simulink model "lab08_3d"  (R2024b)
settings: Solver=ode45  StartTime=0.0  StopTime=15  MaxStep=0.02  MinStep=0.01  RelTol=1e-3
settings Model: Creator=kg53848  LastModifiedBy=kg53848
settings SolverCC: InitialStep=0.01

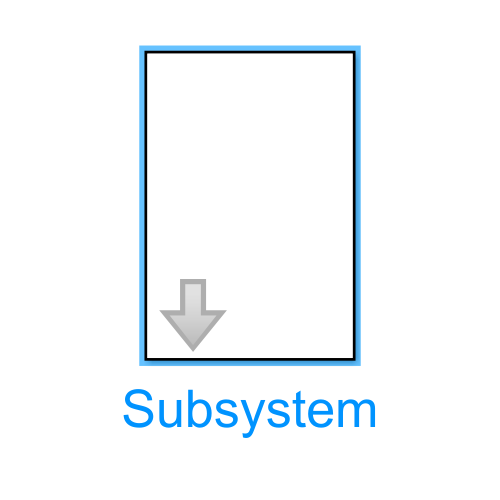
[thumbnail: Simulink's stored preview of the top-level diagram]
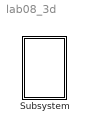
== system lab08_3d ==
  Subsystem : Subsystem  mask{n=3, g=9.81, k=1, m=2, l=4, x=-1, y=-1, xi=[-1 1 1], yi=[1 1 -1], di=[0.1 0.1 0.1], ai=[1 -1 1.5]}
      mask prompts: n "liczba magnesow"; g "przysp ziemskie"; k "wsp tlumienia"; m "m wahadla"; l "l linki dla wahadla"; x "pocz wspolrz wahadla x"; y "pocz wspolrz wahadla y"; xi "polozenie x magnesow"; yi "polozenie y magnesow"; di "odl magnesow od plasz XY"; ai "F magnesow oddz na wahadlo"

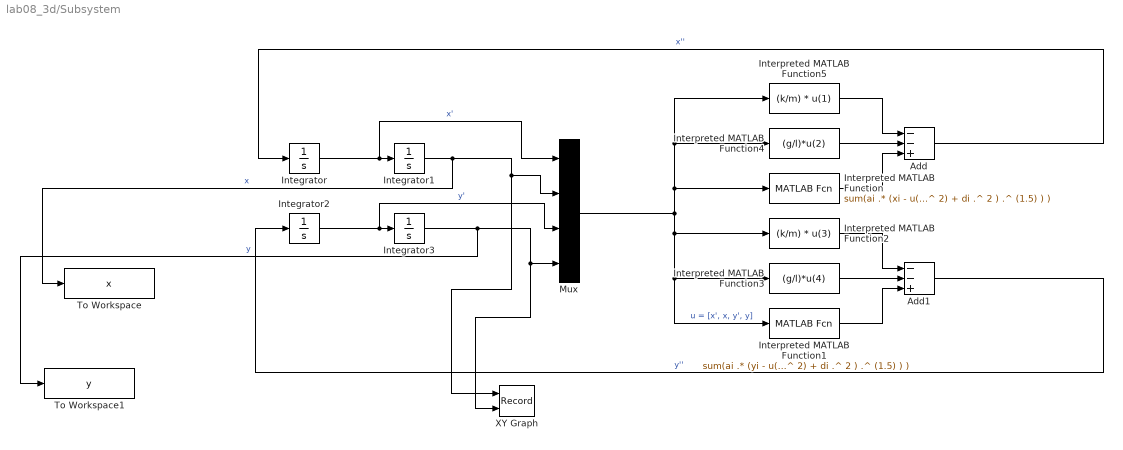
== system lab08_3d/Subsystem ==
  Add : Sum  Inputs=--+
  Add1 : Sum  Inputs=--+
  Integrator : Integrator
  Integrator1 : Integrator  InitialCondition=x
  Integrator2 : Integrator
  Integrator3 : Integrator  InitialCondition=y
  Interpreted MATLAB Function : MATLABFcn  MATLABFcn=sum(ai .* (xi - u(2)) ./ ((((xi-u(2)) .^ 2) + ((yi-u(4)) .^ 2) + di .^ 2 ) .^ (1.5) ) )
  Interpreted MATLAB Function1 : MATLABFcn  MATLABFcn=sum(ai .* (yi - u(4)) ./ ((((xi-u(2)) .^ 2) + ((yi-u(4)) .^ 2) + di .^ 2 ) .^ (1.5) ) )
  Interpreted MATLAB Function2 : MATLABFcn  MATLABFcn=(k/m) * u(3)
  Interpreted MATLAB Function3 : MATLABFcn  MATLABFcn=(g/l)*u(4)
  Interpreted MATLAB Function4 : MATLABFcn  MATLABFcn=(g/l)*u(2)
  Interpreted MATLAB Function5 : MATLABFcn  MATLABFcn=(k/m) * u(1)
  Mux : Mux
  To Workspace : ToWorkspace  VariableName=x  SampleTime=-1
  To Workspace1 : ToWorkspace  VariableName=y  SampleTime=-1
  XY Graph : Record  FileSettingsInternal="{\"entries\":[{\"content\":{\"excelSettings\":{\"content\":{},\"type\":\"Streamout.ExcelSettings\"}},\"type\":\"Streamout.FileSettingStorage\",\"uuid\":\"\"}],\"packageUris\":[\"http:\\/\\/schema.mathworks.com\\/mf0\\/streamout_blocks\\/R2020a\"],\"version\":\"1.0\"}"  Layout=[1 1]  SignalsInternal="{\"entries\":[{\"content\":{\"signals\":[{\"content\":{\"blockPath\":[],\"dimensions\":[1],\"domain\":\"\",\"lineColor\":\"#a2142f\",\"plots\":[ 1 ],\"port\":1,\"sid\":[\"\"],\"signalID\":1,\"signalName\":\"x\"},\"type\":\"RecordBlkView.Signal\",\"uuid\":\"\"},{\"content\":{\"blockPath\":[],\"dimensions\":[1],\"domain\":\"\",\"lineColor\":\"#139fff\",\"plots\":[ 1 ],\"port\":2,\"sid\":[\"\"],\"signalID\":2,\"signalName\":\"y\"},\"type\":\"RecordBlkView.Signal\",\"uuid\":\"\"}]},\"type\":\"RecordBlkView.InputSignals\",\"uuid\":\"\"}],\"packageUris\":[\"http:\\/\\/schema.mathworks.com\\/mf0\\/streamout_blocks\\/R2020a\"],\"version\":\"1.0\"}"  VisualizationBindings="{\"xyplotplugin\":{\"info\":[{\"series\":[{\"bindingParametersList\":[{\"parameter\":\"X-Axis\",\"signalID\":1,\"signalName\":\"x\"},{\"parameter\":\"Y-Axis\",\"signalID\":2,\"signalName\":\"y\"}],\"seriesID\":0}],\"subplotID\":1}]}}"  CompatibilityTag=XY
  wires:
  Mux/1 -> Interpreted MATLAB Function2/1, Interpreted MATLAB Function3/1, Interpreted MATLAB Function1/1, Interpreted MATLAB Function/1, Interpreted MATLAB Function5/1, Interpreted MATLAB Function4/1  "u = [x', x, y', y]"
  Integrator3/1 -> To Workspace1/1, XY Graph/2, Mux/4  "y"
  Interpreted MATLAB Function2/1 -> Add1/1
  Integrator/1 -> Mux/1, Integrator1/1  "x'"
  Integrator2/1 -> Mux/3, Integrator3/1  "y'"
  Add/1 -> Integrator/1  "x''"
  Integrator1/1 -> To Workspace/1, XY Graph/1, Mux/2  "x"
  Add1/1 -> Integrator2/1  "y''"
  Interpreted MATLAB Function5/1 -> Add/1
  Interpreted MATLAB Function4/1 -> Add/2
  Interpreted MATLAB Function1/1 -> Add1/3
  Interpreted MATLAB Function3/1 -> Add1/2
  Interpreted MATLAB Function/1 -> Add/3
